simulink model "ProcessNetworkSimulation"  (R2015b)
settings: Solver=VariableStepAuto  StartTime=0.0  StopTime=1000.0  RelTol=1e-3
libraries: simulink x1, simeventslib x1
(part 18 of 21)

== system ProcessNetworkSimulation/Process_22/Process ==
  OUTQueue : FIFOQueue  Capacity=inf
  ProcessQueue : FIFOQueue  Capacity=Inf  StatAverageWait=on  StatAverageQueueLength=on
      settings: OutputPortMap=o2,o3
  ProcessServer : NServer  NumberOfServers=11  ServiceTimeFrom=Signal port t  StatNumberDeparted=on  StatUtilization=on
      settings: OutputPortMap=o0,o5
  ProcessTime : EventBasedRandomNumber  meanExp=0.05  minUnif=1  meanNorm=2  stdNorm=0.2  Seed=23578
  Routing : EventBasedRandomNumber  Distribution=Arbitrary discrete  valueVecDisc=[0,1,2,3,4,5,6,7,8,9,10,11,12,13,14,15,16,17,18,19,20,21,22,23,24,25,26,27,28,29,30,31,32,33,34,35,36,37,38,39,40,41,42,43]  probVecDisc=[0,0.0298,0.0085,0.0298,0.0383,0.0255,0.0085,0.0383,0.0383,0.0043,0.0298,0.0085,0.0085,0.0383,0.0424,0.0255,0.0085,0.0298,0.0298,0.0298,0.0128,0.0085,0.0085,0.0383,0.0383,0.0085,0.0213,0.0085,0.0298,0.0213,0.0085,0.034,0.0383,0.0383,0.0255,0.0128,0.0213,0.0298,0.0213,0.0128,0.0085,0.0383,0.0426,0]  Seed=26795
  read_ProcessTimer : ReadTimer  TimerTag=T_Process_22  StatAverageTimeElapsed=on
      settings: OutputPortMap=o3
  setRouting : SetAttribute  AttributeName=outputFlowNode  AttributeFrom=Signal port  EvaluatedAttributeValue={ []}
  start_ProcessTimer : StartTimer  TimerTag=T_Process_22  TimerStartedOption=Restart
  IN_Job : PMIOPort  Port=1  Side=Left
  OUT_Job : PMIOPort  Port=2  Side=Right
  wires:
  Routing/1 -> setRouting/1
  ProcessTime/1 -> ProcessServer/1
  connections:
  setRouting/LConn1 -- OUTQueue/RConn1
  IN_Job/RConn1 -- start_ProcessTimer/LConn1
  ProcessServer/RConn1 -- read_ProcessTimer/LConn1
  start_ProcessTimer/RConn1 -- ProcessQueue/LConn1
  ProcessQueue/RConn1 -- ProcessServer/LConn1
  read_ProcessTimer/RConn1 -- OUTQueue/LConn1
  OUT_Job/RConn1 -- setRouting/RConn1

== system ProcessNetworkSimulation/Process_23/Process ==
  OUTQueue : FIFOQueue  Capacity=inf
  ProcessQueue : FIFOQueue  Capacity=Inf  StatAverageWait=on  StatAverageQueueLength=on
      settings: OutputPortMap=o2,o3
  ProcessServer : NServer  NumberOfServers=12  ServiceTimeFrom=Signal port t  StatNumberDeparted=on  StatUtilization=on
      settings: OutputPortMap=o0,o5
  ProcessTime : EventBasedRandomNumber  meanExp=0.05  minUnif=1  meanNorm=2  stdNorm=0.2  Seed=30012
  Routing : EventBasedRandomNumber  Distribution=Arbitrary discrete  valueVecDisc=[0,1,2,3,4,5,6,7,8,9,10,11,12,13,14,15,16,17,18,19,20,21,22,23,24,25,26,27,28,29,30,31,32,33,34,35,36]  probVecDisc=[0,0.0413,0.0229,0.0275,0.0275,0.0092,0.0413,0.0458,0.0275,0.0321,0.0413,0.0413,0.0138,0.0367,0.0092,0.0092,0.0275,0.0413,0.0046,0.0413,0.0138,0.0229,0.0275,0.0092,0.0092,0.0275,0.0413,0.0275,0.0459,0.0459,0.0229,0.0413,0.0275,0.0275,0.0321,0.0321,0.0046]  Seed=33229
  read_ProcessTimer : ReadTimer  TimerTag=T_Process_23  StatAverageTimeElapsed=on
      settings: OutputPortMap=o3
  setRouting : SetAttribute  AttributeName=outputFlowNode  AttributeFrom=Signal port  EvaluatedAttributeValue={ []}
  start_ProcessTimer : StartTimer  TimerTag=T_Process_23  TimerStartedOption=Restart
  IN_Job : PMIOPort  Port=1  Side=Left
  OUT_Job : PMIOPort  Port=2  Side=Right
  wires:
  Routing/1 -> setRouting/1
  ProcessTime/1 -> ProcessServer/1
  connections:
  setRouting/LConn1 -- OUTQueue/RConn1
  IN_Job/RConn1 -- start_ProcessTimer/LConn1
  ProcessServer/RConn1 -- read_ProcessTimer/LConn1
  start_ProcessTimer/RConn1 -- ProcessQueue/LConn1
  ProcessQueue/RConn1 -- ProcessServer/LConn1
  read_ProcessTimer/RConn1 -- OUTQueue/LConn1
  OUT_Job/RConn1 -- setRouting/RConn1

== system ProcessNetworkSimulation/Process_24/Process ==
  OUTQueue : FIFOQueue  Capacity=inf
  ProcessQueue : FIFOQueue  Capacity=Inf  StatAverageWait=on  StatAverageQueueLength=on
      settings: OutputPortMap=o2,o3
  ProcessServer : NServer  NumberOfServers=12  ServiceTimeFrom=Signal port t  StatNumberDeparted=on  StatUtilization=on
      settings: OutputPortMap=o0,o5
  ProcessTime : EventBasedRandomNumber  meanExp=0.05  minUnif=1  meanNorm=2  stdNorm=0.2  Seed=36446
  Routing : EventBasedRandomNumber  Distribution=Arbitrary discrete  valueVecDisc=[0,1,2,3,4,5,6,7,8,9,10,11,12,13,14,15,16,17,18,19,20,21,22,23,24,25,26,27,28,29,30,31,32,33,34,35,36]  probVecDisc=[0,0.0051,0.0455,0.0152,0.0051,0.0253,0.0455,0.0354,0.0101,0.0152,0.0354,0.0455,0.0101,0.0354,0.0455,0.0152,0.0101,0.0303,0.0051,0.0101,0.0455,0.0455,0.0354,0.0494,0.0455,0.0455,0.0101,0.0253,0.0354,0.0303,0.0404,0.0354,0.0404,0.0303,0.0051,0.0354,0]  Seed=39663
  read_ProcessTimer : ReadTimer  TimerTag=T_Process_24  StatAverageTimeElapsed=on
      settings: OutputPortMap=o3
  setRouting : SetAttribute  AttributeName=outputFlowNode  AttributeFrom=Signal port  EvaluatedAttributeValue={ []}
  start_ProcessTimer : StartTimer  TimerTag=T_Process_24  TimerStartedOption=Restart
  IN_Job : PMIOPort  Port=1  Side=Left
  OUT_Job : PMIOPort  Port=2  Side=Right
  wires:
  Routing/1 -> setRouting/1
  ProcessTime/1 -> ProcessServer/1
  connections:
  setRouting/LConn1 -- OUTQueue/RConn1
  IN_Job/RConn1 -- start_ProcessTimer/LConn1
  ProcessServer/RConn1 -- read_ProcessTimer/LConn1
  start_ProcessTimer/RConn1 -- ProcessQueue/LConn1
  ProcessQueue/RConn1 -- ProcessServer/LConn1
  read_ProcessTimer/RConn1 -- OUTQueue/LConn1
  OUT_Job/RConn1 -- setRouting/RConn1

== system ProcessNetworkSimulation/Process_25/Process ==
  OUTQueue : FIFOQueue  Capacity=inf
  ProcessQueue : FIFOQueue  Capacity=Inf  StatAverageWait=on  StatAverageQueueLength=on
      settings: OutputPortMap=o2,o3
  ProcessServer : NServer  NumberOfServers=11  ServiceTimeFrom=Signal port t  StatNumberDeparted=on  StatUtilization=on
      settings: OutputPortMap=o0,o5
  ProcessTime : EventBasedRandomNumber  meanExp=0.05  minUnif=1  meanNorm=2  stdNorm=0.2  Seed=42880
  Routing : EventBasedRandomNumber  Distribution=Arbitrary discrete  valueVecDisc=[0,1,2,3,4,5,6,7,8,9,10,11,12,13,14,15,16,17,18,19,20,21,22,23,24,25,26,27,28,29,30,31,32,33,34,35,36,37,38,39,40,41]  probVecDisc=[0,0.0323,0.023,0.0092,0.0092,0.0415,0.023,0.0046,0.0462,0.0092,0.0461,0.0092,0.023,0.0323,0.0323,0.0323,0.0138,0.0092,0.0415,0.0138,0.0415,0.0092,0.0276,0.023,0.0323,0.023,0.0415,0.0092,0.0415,0.0046,0.0461,0.0415,0.0369,0.023,0.023,0.023,0.0046,0.0461,0.0323,0.0092,0.0092,0]  Seed=46097
  read_ProcessTimer : ReadTimer  TimerTag=T_Process_25  StatAverageTimeElapsed=on
      settings: OutputPortMap=o3
  setRouting : SetAttribute  AttributeName=outputFlowNode  AttributeFrom=Signal port  EvaluatedAttributeValue={ []}
  start_ProcessTimer : StartTimer  TimerTag=T_Process_25  TimerStartedOption=Restart
  IN_Job : PMIOPort  Port=1  Side=Left
  OUT_Job : PMIOPort  Port=2  Side=Right
  wires:
  Routing/1 -> setRouting/1
  ProcessTime/1 -> ProcessServer/1
  connections:
  setRouting/LConn1 -- OUTQueue/RConn1
  IN_Job/RConn1 -- start_ProcessTimer/LConn1
  ProcessServer/RConn1 -- read_ProcessTimer/LConn1
  start_ProcessTimer/RConn1 -- ProcessQueue/LConn1
  ProcessQueue/RConn1 -- ProcessServer/LConn1
  read_ProcessTimer/RConn1 -- OUTQueue/LConn1
  OUT_Job/RConn1 -- setRouting/RConn1

== system ProcessNetworkSimulation/Process_26/Process ==
  OUTQueue : FIFOQueue  Capacity=inf
  ProcessQueue : FIFOQueue  Capacity=Inf  StatAverageWait=on  StatAverageQueueLength=on
      settings: OutputPortMap=o2,o3
  ProcessServer : NServer  NumberOfServers=12  ServiceTimeFrom=Signal port t  StatNumberDeparted=on  StatUtilization=on
      settings: OutputPortMap=o0,o5
  ProcessTime : EventBasedRandomNumber  meanExp=0.05  minUnif=1  meanNorm=2  stdNorm=0.2  Seed=49314
  Routing : EventBasedRandomNumber  Distribution=Arbitrary discrete  valueVecDisc=[0,1,2,3,4,5,6,7,8,9,10,11,12,13,14,15,16,17,18,19,20,21,22,23,24,25,26,27,28,29,30,31,32,33,34,35,36,37,38,39,40]  probVecDisc=[0,0.0457,0.0406,0.0152,0.0102,0.0102,0.0102,0.0102,0.0254,0.0457,0.0499,0.0355,0.0102,0.0102,0.0406,0.0102,0.0355,0.0051,0.0457,0.0102,0.0152,0.0051,0.0254,0.0457,0.0102,0.0406,0.0305,0.0508,0.0457,0.0254,0.0102,0.0051,0.0355,0.0102,0.0305,0.0102,0.0102,0.0457,0.0102,0.0254,0.0457]  Seed=52531
  read_ProcessTimer : ReadTimer  TimerTag=T_Process_26  StatAverageTimeElapsed=on
      settings: OutputPortMap=o3
  setRouting : SetAttribute  AttributeName=outputFlowNode  AttributeFrom=Signal port  EvaluatedAttributeValue={ []}
  start_ProcessTimer : StartTimer  TimerTag=T_Process_26  TimerStartedOption=Restart
  IN_Job : PMIOPort  Port=1  Side=Left
  OUT_Job : PMIOPort  Port=2  Side=Right
  wires:
  Routing/1 -> setRouting/1
  ProcessTime/1 -> ProcessServer/1
  connections:
  setRouting/LConn1 -- OUTQueue/RConn1
  IN_Job/RConn1 -- start_ProcessTimer/LConn1
  ProcessServer/RConn1 -- read_ProcessTimer/LConn1
  start_ProcessTimer/RConn1 -- ProcessQueue/LConn1
  ProcessQueue/RConn1 -- ProcessServer/LConn1
  read_ProcessTimer/RConn1 -- OUTQueue/LConn1
  OUT_Job/RConn1 -- setRouting/RConn1

== system ProcessNetworkSimulation/Process_27/Process ==
  OUTQueue : FIFOQueue  Capacity=inf
  ProcessQueue : FIFOQueue  Capacity=Inf  StatAverageWait=on  StatAverageQueueLength=on
      settings: OutputPortMap=o2,o3
  ProcessServer : NServer  NumberOfServers=14  ServiceTimeFrom=Signal port t  StatNumberDeparted=on  StatUtilization=on
      settings: OutputPortMap=o0,o5
  ProcessTime : EventBasedRandomNumber  meanExp=0.05  minUnif=1  meanNorm=2  stdNorm=0.2  Seed=55748
  Routing : EventBasedRandomNumber  Distribution=Arbitrary discrete  valueVecDisc=[0,1,2,3,4,5,6,7,8,9,10,11,12,13,14,15,16,17,18,19,20,21,22,23,24,25,26,27,28,29,30,31,32,33,34,35,36,37,38,39,40,41,42,43]  probVecDisc=[0,0.0353,0.0353,0.0078,0.0078,0.0078,0.0196,0.0275,0.0078,0.0275,0.0353,0.0275,0.0353,0.0275,0.0196,0.0196,0.0235,0.0275,0.0275,0.0353,0.0275,0.0353,0.0118,0.0353,0.0078,0.0275,0.0353,0.0275,0.0078,0.039,0.0235,0.0235,0.0118,0.0275,0.0118,0.0235,0.0275,0.0196,0.0314,0.0235,0.0235,0.0353,0.0078,0]  Seed=58965
  read_ProcessTimer : ReadTimer  TimerTag=T_Process_27  StatAverageTimeElapsed=on
      settings: OutputPortMap=o3
  setRouting : SetAttribute  AttributeName=outputFlowNode  AttributeFrom=Signal port  EvaluatedAttributeValue={ []}
  start_ProcessTimer : StartTimer  TimerTag=T_Process_27  TimerStartedOption=Restart
  IN_Job : PMIOPort  Port=1  Side=Left
  OUT_Job : PMIOPort  Port=2  Side=Right
  wires:
  Routing/1 -> setRouting/1
  ProcessTime/1 -> ProcessServer/1
  connections:
  setRouting/LConn1 -- OUTQueue/RConn1
  IN_Job/RConn1 -- start_ProcessTimer/LConn1
  ProcessServer/RConn1 -- read_ProcessTimer/LConn1
  start_ProcessTimer/RConn1 -- ProcessQueue/LConn1
  ProcessQueue/RConn1 -- ProcessServer/LConn1
  read_ProcessTimer/RConn1 -- OUTQueue/LConn1
  OUT_Job/RConn1 -- setRouting/RConn1

== system ProcessNetworkSimulation/Process_28/Process ==
  OUTQueue : FIFOQueue  Capacity=inf
  ProcessQueue : FIFOQueue  Capacity=Inf  StatAverageWait=on  StatAverageQueueLength=on
      settings: OutputPortMap=o2,o3
  ProcessServer : NServer  NumberOfServers=8  ServiceTimeFrom=Signal port t  StatNumberDeparted=on  StatUtilization=on
      settings: OutputPortMap=o0,o5
  ProcessTime : EventBasedRandomNumber  meanExp=0.05  minUnif=1  meanNorm=2  stdNorm=0.2  Seed=62182
  Routing : EventBasedRandomNumber  Distribution=Arbitrary discrete  valueVecDisc=[0,1,2,3,4,5,6,7,8,9,10,11,12,13,14,15,16,17,18,19,20,21,22,23,24,25,26,27,28,29]  probVecDisc=[0,0.0643,0.0143,0.0143,0.0143,0.05,0.05,0.0571,0.0571,0.0643,0.0143,0.0715,0.0357,0.05,0.0214,0.0143,0.0357,0.0643,0.0643,0.0071,0.0429,0.0357,0.0143,0.0357,0.0214,0.05,0.0143,0.0143,0.0071,0]  Seed=65399
  read_ProcessTimer : ReadTimer  TimerTag=T_Process_28  StatAverageTimeElapsed=on
      settings: OutputPortMap=o3
  setRouting : SetAttribute  AttributeName=outputFlowNode  AttributeFrom=Signal port  EvaluatedAttributeValue={ []}
  start_ProcessTimer : StartTimer  TimerTag=T_Process_28  TimerStartedOption=Restart
  IN_Job : PMIOPort  Port=1  Side=Left
  OUT_Job : PMIOPort  Port=2  Side=Right
  wires:
  Routing/1 -> setRouting/1
  ProcessTime/1 -> ProcessServer/1
  connections:
  setRouting/LConn1 -- OUTQueue/RConn1
  IN_Job/RConn1 -- start_ProcessTimer/LConn1
  ProcessServer/RConn1 -- read_ProcessTimer/LConn1
  start_ProcessTimer/RConn1 -- ProcessQueue/LConn1
  ProcessQueue/RConn1 -- ProcessServer/LConn1
  read_ProcessTimer/RConn1 -- OUTQueue/LConn1
  OUT_Job/RConn1 -- setRouting/RConn1

== system ProcessNetworkSimulation/Process_29/Process ==
  OUTQueue : FIFOQueue  Capacity=inf
  ProcessQueue : FIFOQueue  Capacity=Inf  StatAverageWait=on  StatAverageQueueLength=on
      settings: OutputPortMap=o2,o3
  ProcessServer : NServer  NumberOfServers=12  ServiceTimeFrom=Signal port t  StatNumberDeparted=on  StatUtilization=on
      settings: OutputPortMap=o0,o5
  ProcessTime : EventBasedRandomNumber  meanExp=0.05  minUnif=1  meanNorm=2  stdNorm=0.2  Seed=3080
  Routing : EventBasedRandomNumber  Distribution=Arbitrary discrete  valueVecDisc=[0,1,2,3,4,5,6,7,8,9,10,11,12,13,14,15,16,17,18,19,20,21,22,23,24,25,26,27,28,29,30,31,32,33,34,35,36,37]  probVecDisc=[0,0.0142,0.0142,0.033,0.0283,0.0425,0.0094,0.0377,0.0471,0.033,0.0047,0.0047,0.0283,0.0283,0.0377,0.0425,0.0047,0.033,0.0094,0.0425,0.0425,0.0094,0.0472,0.0283,0.0283,0.0377,0.0283,0.033,0.0236,0.033,0.0283,0.0425,0.0425,0.0142,0.0094,0.0094,0.0472,0]  Seed=6297
  read_ProcessTimer : ReadTimer  TimerTag=T_Process_29  StatAverageTimeElapsed=on
      settings: OutputPortMap=o3
  setRouting : SetAttribute  AttributeName=outputFlowNode  AttributeFrom=Signal port  EvaluatedAttributeValue={ []}
  start_ProcessTimer : StartTimer  TimerTag=T_Process_29  TimerStartedOption=Restart
  IN_Job : PMIOPort  Port=1  Side=Left
  OUT_Job : PMIOPort  Port=2  Side=Right
  wires:
  Routing/1 -> setRouting/1
  ProcessTime/1 -> ProcessServer/1
  connections:
  setRouting/LConn1 -- OUTQueue/RConn1
  IN_Job/RConn1 -- start_ProcessTimer/LConn1
  ProcessServer/RConn1 -- read_ProcessTimer/LConn1
  start_ProcessTimer/RConn1 -- ProcessQueue/LConn1
  ProcessQueue/RConn1 -- ProcessServer/LConn1
  read_ProcessTimer/RConn1 -- OUTQueue/LConn1
  OUT_Job/RConn1 -- setRouting/RConn1

== system ProcessNetworkSimulation/Process_3/Process ==
  OUTQueue : FIFOQueue  Capacity=inf
  ProcessQueue : FIFOQueue  Capacity=Inf  StatAverageWait=on  StatAverageQueueLength=on
      settings: OutputPortMap=o2,o3
  ProcessServer : NServer  NumberOfServers=10  ServiceTimeFrom=Signal port t  StatNumberDeparted=on  StatUtilization=on
      settings: OutputPortMap=o0,o5
  ProcessTime : EventBasedRandomNumber  meanExp=0.05  minUnif=1  meanNorm=2  stdNorm=0.2  Seed=9514
  Routing : EventBasedRandomNumber  Distribution=Arbitrary discrete  valueVecDisc=[0,1,2,3,4,5,6,7,8,9,10,11,12,13,14,15,16,17,18,19,20,21,22,23,24,25,26,27,28,29,30,31]  probVecDisc=[0,0.0335,0.0503,0.0503,0.0112,0.0279,0.0279,0.0503,0.0503,0.0112,0.0391,0.0557,0.0391,0.0112,0.0168,0.0503,0.0335,0.0391,0.0112,0.0335,0.0112,0.0391,0.0056,0.0279,0.0112,0.0279,0.0503,0.0503,0.0391,0.0559,0.0112,0.0279]  Seed=12731
  read_ProcessTimer : ReadTimer  TimerTag=T_Process_3  StatAverageTimeElapsed=on
      settings: OutputPortMap=o3
  setRouting : SetAttribute  AttributeName=outputFlowNode  AttributeFrom=Signal port  EvaluatedAttributeValue={ []}
  start_ProcessTimer : StartTimer  TimerTag=T_Process_3  TimerStartedOption=Restart
  IN_Job : PMIOPort  Port=1  Side=Left
  OUT_Job : PMIOPort  Port=2  Side=Right
  wires:
  Routing/1 -> setRouting/1
  ProcessTime/1 -> ProcessServer/1
  connections:
  setRouting/LConn1 -- OUTQueue/RConn1
  IN_Job/RConn1 -- start_ProcessTimer/LConn1
  ProcessServer/RConn1 -- read_ProcessTimer/LConn1
  start_ProcessTimer/RConn1 -- ProcessQueue/LConn1
  ProcessQueue/RConn1 -- ProcessServer/LConn1
  read_ProcessTimer/RConn1 -- OUTQueue/LConn1
  OUT_Job/RConn1 -- setRouting/RConn1

== system ProcessNetworkSimulation/Process_30/Process ==
  OUTQueue : FIFOQueue  Capacity=inf
  ProcessQueue : FIFOQueue  Capacity=Inf  StatAverageWait=on  StatAverageQueueLength=on
      settings: OutputPortMap=o2,o3
  ProcessServer : NServer  NumberOfServers=12  ServiceTimeFrom=Signal port t  StatNumberDeparted=on  StatUtilization=on
      settings: OutputPortMap=o0,o5
  ProcessTime : EventBasedRandomNumber  meanExp=0.05  minUnif=1  meanNorm=2  stdNorm=0.2  Seed=15948
  Routing : EventBasedRandomNumber  Distribution=Arbitrary discrete  valueVecDisc=[0,1,2,3,4,5,6,7,8,9,10,11,12,13,14,15,16,17,18,19,20,21,22,23,24,25,26,27,28,29,30,31,32,33,34,35,36,37,38]  probVecDisc=[0,0.0474,0.0316,0.0316,0.0316,0.0158,0.0527,0.0421,0.0368,0.0105,0.0316,0.0105,0.0474,0.0263,0.0316,0.0105,0.0368,0.0053,0.0158,0.0053,0.0474,0.0368,0.0105,0.0474,0.0053,0.0316,0.0105,0.0053,0.0105,0.0158,0.0526,0.0105,0.0368,0.0105,0.0263,0.0368,0.0474,0.0368,0]  Seed=19165
  read_ProcessTimer : ReadTimer  TimerTag=T_Process_30  StatAverageTimeElapsed=on
      settings: OutputPortMap=o3
  setRouting : SetAttribute  AttributeName=outputFlowNode  AttributeFrom=Signal port  EvaluatedAttributeValue={ []}
  start_ProcessTimer : StartTimer  TimerTag=T_Process_30  TimerStartedOption=Restart
  IN_Job : PMIOPort  Port=1  Side=Left
  OUT_Job : PMIOPort  Port=2  Side=Right
  wires:
  Routing/1 -> setRouting/1
  ProcessTime/1 -> ProcessServer/1
  connections:
  setRouting/LConn1 -- OUTQueue/RConn1
  IN_Job/RConn1 -- start_ProcessTimer/LConn1
  ProcessServer/RConn1 -- read_ProcessTimer/LConn1
  start_ProcessTimer/RConn1 -- ProcessQueue/LConn1
  ProcessQueue/RConn1 -- ProcessServer/LConn1
  read_ProcessTimer/RConn1 -- OUTQueue/LConn1
  OUT_Job/RConn1 -- setRouting/RConn1

== system ProcessNetworkSimulation/Process_31/Process ==
  OUTQueue : FIFOQueue  Capacity=inf
  ProcessQueue : FIFOQueue  Capacity=Inf  StatAverageWait=on  StatAverageQueueLength=on
      settings: OutputPortMap=o2,o3
  ProcessServer : NServer  NumberOfServers=9  ServiceTimeFrom=Signal port t  StatNumberDeparted=on  StatUtilization=on
      settings: OutputPortMap=o0,o5
  ProcessTime : EventBasedRandomNumber  meanExp=0.05  minUnif=1  meanNorm=2  stdNorm=0.2  Seed=22382
  Routing : EventBasedRandomNumber  Distribution=Arbitrary discrete  valueVecDisc=[0,1,2,3,4,5,6,7,8,9,10,11,12,13,14,15,16,17,18,19,20,21,22,23,24,25,26,27,28]  probVecDisc=[0,0.0071,0.0142,0.0496,0.0638,0.0638,0.0355,0.0142,0.0496,0.0426,0.0071,0.0355,0.0638,0.0426,0.0426,0.0707,0.0638,0.0213,0.0142,0.0213,0.0213,0.0071,0.0142,0.0071,0.0426,0.0426,0.0638,0.0142,0.0638]  Seed=25599
  read_ProcessTimer : ReadTimer  TimerTag=T_Process_31  StatAverageTimeElapsed=on
      settings: OutputPortMap=o3
  setRouting : SetAttribute  AttributeName=outputFlowNode  AttributeFrom=Signal port  EvaluatedAttributeValue={ []}
  start_ProcessTimer : StartTimer  TimerTag=T_Process_31  TimerStartedOption=Restart
  IN_Job : PMIOPort  Port=1  Side=Left
  OUT_Job : PMIOPort  Port=2  Side=Right
  wires:
  Routing/1 -> setRouting/1
  ProcessTime/1 -> ProcessServer/1
  connections:
  setRouting/LConn1 -- OUTQueue/RConn1
  IN_Job/RConn1 -- start_ProcessTimer/LConn1
  ProcessServer/RConn1 -- read_ProcessTimer/LConn1
  start_ProcessTimer/RConn1 -- ProcessQueue/LConn1
  ProcessQueue/RConn1 -- ProcessServer/LConn1
  read_ProcessTimer/RConn1 -- OUTQueue/LConn1
  OUT_Job/RConn1 -- setRouting/RConn1

== system ProcessNetworkSimulation/Process_32/Process ==
  OUTQueue : FIFOQueue  Capacity=inf
  ProcessQueue : FIFOQueue  Capacity=Inf  StatAverageWait=on  StatAverageQueueLength=on
      settings: OutputPortMap=o2,o3
  ProcessServer : NServer  NumberOfServers=10  ServiceTimeFrom=Signal port t  StatNumberDeparted=on  StatUtilization=on
      settings: OutputPortMap=o0,o5
  ProcessTime : EventBasedRandomNumber  meanExp=0.05  minUnif=1  meanNorm=2  stdNorm=0.2  Seed=28816
  Routing : EventBasedRandomNumber  Distribution=Arbitrary discrete  valueVecDisc=[0,1,2,3,4,5,6,7,8,9,10,11,12,13,14,15,16,17,18,19,20,21,22,23,24,25,26,27,28,29,30,31,32,33,34,35,36,37,38]  probVecDisc=[0,0.0114,0.0284,0.0564,0.0114,0.0398,0.0284,0.0284,0.0114,0.0114,0.0114,0.017,0.0284,0.0398,0.0114,0.0455,0.0511,0.0284,0.0398,0.0398,0.0114,0.0398,0.0511,0.0114,0.0114,0.0284,0.0114,0.0284,0.017,0.0398,0.0284,0.0114,0.0398,0.0341,0.0284,0.0114,0.0398,0.017,0]  Seed=32033
  read_ProcessTimer : ReadTimer  TimerTag=T_Process_32  StatAverageTimeElapsed=on
      settings: OutputPortMap=o3
  setRouting : SetAttribute  AttributeName=outputFlowNode  AttributeFrom=Signal port  EvaluatedAttributeValue={ []}
  start_ProcessTimer : StartTimer  TimerTag=T_Process_32  TimerStartedOption=Restart
  IN_Job : PMIOPort  Port=1  Side=Left
  OUT_Job : PMIOPort  Port=2  Side=Right
  wires:
  Routing/1 -> setRouting/1
  ProcessTime/1 -> ProcessServer/1
  connections:
  setRouting/LConn1 -- OUTQueue/RConn1
  IN_Job/RConn1 -- start_ProcessTimer/LConn1
  ProcessServer/RConn1 -- read_ProcessTimer/LConn1
  start_ProcessTimer/RConn1 -- ProcessQueue/LConn1
  ProcessQueue/RConn1 -- ProcessServer/LConn1
  read_ProcessTimer/RConn1 -- OUTQueue/LConn1
  OUT_Job/RConn1 -- setRouting/RConn1

== system ProcessNetworkSimulation/Process_33/Process ==
  OUTQueue : FIFOQueue  Capacity=inf
  ProcessQueue : FIFOQueue  Capacity=Inf  StatAverageWait=on  StatAverageQueueLength=on
      settings: OutputPortMap=o2,o3
  ProcessServer : NServer  NumberOfServers=11  ServiceTimeFrom=Signal port t  StatNumberDeparted=on  StatUtilization=on
      settings: OutputPortMap=o0,o5
  ProcessTime : EventBasedRandomNumber  meanExp=0.05  minUnif=1  meanNorm=2  stdNorm=0.2  Seed=35250
  Routing : EventBasedRandomNumber  Distribution=Arbitrary discrete  valueVecDisc=[0,1,2,3,4,5,6,7,8,9,10,11,12,13,14,15,16,17,18,19,20,21,22,23,24,25,26,27,28,29,30,31,32,33,34,35,36,37,38,39,40,41,42]  probVecDisc=[0,0.0101,0.0446,0.0151,0.0452,0.0452,0.0101,0.0452,0.0101,0.0151,0.0452,0.0452,0.0251,0.0352,0.0101,0.0151,0.0352,0.0151,0.0352,0.0302,0.0352,0.0101,0.005,0.0101,0.0452,0.0101,0.0251,0.0101,0.0101,0.0302,0.0251,0.0251,0.0452,0.0101,0.005,0.0101,0.0101,0.0101,0.0251,0.0302,0.0452,0.0352,0]  Seed=38467
  read_ProcessTimer : ReadTimer  TimerTag=T_Process_33  StatAverageTimeElapsed=on
      settings: OutputPortMap=o3
  setRouting : SetAttribute  AttributeName=outputFlowNode  AttributeFrom=Signal port  EvaluatedAttributeValue={ []}
  start_ProcessTimer : StartTimer  TimerTag=T_Process_33  TimerStartedOption=Restart
  IN_Job : PMIOPort  Port=1  Side=Left
  OUT_Job : PMIOPort  Port=2  Side=Right
  wires:
  Routing/1 -> setRouting/1
  ProcessTime/1 -> ProcessServer/1
  connections:
  setRouting/LConn1 -- OUTQueue/RConn1
  IN_Job/RConn1 -- start_ProcessTimer/LConn1
  ProcessServer/RConn1 -- read_ProcessTimer/LConn1
  start_ProcessTimer/RConn1 -- ProcessQueue/LConn1
  ProcessQueue/RConn1 -- ProcessServer/LConn1
  read_ProcessTimer/RConn1 -- OUTQueue/LConn1
  OUT_Job/RConn1 -- setRouting/RConn1

== system ProcessNetworkSimulation/Process_34/Process ==
  OUTQueue : FIFOQueue  Capacity=inf
  ProcessQueue : FIFOQueue  Capacity=Inf  StatAverageWait=on  StatAverageQueueLength=on
      settings: OutputPortMap=o2,o3
  ProcessServer : NServer  NumberOfServers=11  ServiceTimeFrom=Signal port t  StatNumberDeparted=on  StatUtilization=on
      settings: OutputPortMap=o0,o5
  ProcessTime : EventBasedRandomNumber  meanExp=0.05  minUnif=1  meanNorm=2  stdNorm=0.2  Seed=41684
  Routing : EventBasedRandomNumber  Distribution=Arbitrary discrete  valueVecDisc=[0,1,2,3,4,5,6,7,8,9,10,11,12,13,14,15,16,17,18,19,20,21,22,23,24,25,26,27,28,29,30,31,32,33,34,35,36,37,38,39,40]  probVecDisc=[0,0.0259,0.0129,0.0302,0.0086,0.0216,0.0129,0.0302,0.0129,0.0345,0.0345,0.0388,0.0259,0.0216,0.0302,0.0086,0.0216,0.0086,0.0086,0.0302,0.0424,0.0259,0.0388,0.0259,0.0302,0.0302,0.0086,0.0259,0.0388,0.0302,0.0216,0.0129,0.0216,0.0302,0.0216,0.0259,0.0302,0.0431,0.0216,0.0259,0.0302]  Seed=44901
  read_ProcessTimer : ReadTimer  TimerTag=T_Process_34  StatAverageTimeElapsed=on
      settings: OutputPortMap=o3
  setRouting : SetAttribute  AttributeName=outputFlowNode  AttributeFrom=Signal port  EvaluatedAttributeValue={ []}
  start_ProcessTimer : StartTimer  TimerTag=T_Process_34  TimerStartedOption=Restart
  IN_Job : PMIOPort  Port=1  Side=Left
  OUT_Job : PMIOPort  Port=2  Side=Right
  wires:
  Routing/1 -> setRouting/1
  ProcessTime/1 -> ProcessServer/1
  connections:
  setRouting/LConn1 -- OUTQueue/RConn1
  IN_Job/RConn1 -- start_ProcessTimer/LConn1
  ProcessServer/RConn1 -- read_ProcessTimer/LConn1
  start_ProcessTimer/RConn1 -- ProcessQueue/LConn1
  ProcessQueue/RConn1 -- ProcessServer/LConn1
  read_ProcessTimer/RConn1 -- OUTQueue/LConn1
  OUT_Job/RConn1 -- setRouting/RConn1

== system ProcessNetworkSimulation/Process_35/Process ==
  OUTQueue : FIFOQueue  Capacity=inf
  ProcessQueue : FIFOQueue  Capacity=Inf  StatAverageWait=on  StatAverageQueueLength=on
      settings: OutputPortMap=o2,o3
  ProcessServer : NServer  NumberOfServers=12  ServiceTimeFrom=Signal port t  StatNumberDeparted=on  StatUtilization=on
      settings: OutputPortMap=o0,o5
  ProcessTime : EventBasedRandomNumber  meanExp=0.05  minUnif=1  meanNorm=2  stdNorm=0.2  Seed=48118
  Routing : EventBasedRandomNumber  Distribution=Arbitrary discrete  valueVecDisc=[0,1,2,3,4,5,6,7,8,9,10,11,12,13,14,15,16,17,18,19,20,21,22,23,24,25,26,27,28,29,30,31,32,33,34,35,36,37,38]  probVecDisc=[0,0.0133,0.04,0.0311,0.0222,0.04,0.0089,0.04,0.0445,0.0089,0.0267,0.0267,0.0222,0.0222,0.0089,0.0267,0.0089,0.04,0.0133,0.04,0.0222,0.0089,0.0267,0.0089,0.0089,0.0267,0.0133,0.0222,0.0444,0.0444,0.04,0.0222,0.0222,0.0267,0.0356,0.0311,0.0311,0.04,0.04]  Seed=51335
  read_ProcessTimer : ReadTimer  TimerTag=T_Process_35  StatAverageTimeElapsed=on
      settings: OutputPortMap=o3
  setRouting : SetAttribute  AttributeName=outputFlowNode  AttributeFrom=Signal port  EvaluatedAttributeValue={ []}
  start_ProcessTimer : StartTimer  TimerTag=T_Process_35  TimerStartedOption=Restart
  IN_Job : PMIOPort  Port=1  Side=Left
  OUT_Job : PMIOPort  Port=2  Side=Right
  wires:
  Routing/1 -> setRouting/1
  ProcessTime/1 -> ProcessServer/1
  connections:
  setRouting/LConn1 -- OUTQueue/RConn1
  IN_Job/RConn1 -- start_ProcessTimer/LConn1
  ProcessServer/RConn1 -- read_ProcessTimer/LConn1
  start_ProcessTimer/RConn1 -- ProcessQueue/LConn1
  ProcessQueue/RConn1 -- ProcessServer/LConn1
  read_ProcessTimer/RConn1 -- OUTQueue/LConn1
  OUT_Job/RConn1 -- setRouting/RConn1

== system ProcessNetworkSimulation/Process_36/Process ==
  OUTQueue : FIFOQueue  Capacity=inf
  ProcessQueue : FIFOQueue  Capacity=Inf  StatAverageWait=on  StatAverageQueueLength=on
      settings: OutputPortMap=o2,o3
  ProcessServer : NServer  NumberOfServers=11  ServiceTimeFrom=Signal port t  StatNumberDeparted=on  StatUtilization=on
      settings: OutputPortMap=o0,o5
  ProcessTime : EventBasedRandomNumber  meanExp=0.05  minUnif=1  meanNorm=2  stdNorm=0.2  Seed=54552
  Routing : EventBasedRandomNumber  Distribution=Arbitrary discrete  valueVecDisc=[0,1,2,3,4,5,6,7,8,9,10,11,12,13,14,15,16,17,18,19,20,21,22,23,24,25,26,27,28,29,30,31,32,33,34,35,36]  probVecDisc=[0,0.0374,0.0107,0.0321,0.0267,0.0374,0.0428,0.0267,0.0107,0.0374,0.0321,0.0374,0.0539,0.0321,0.016,0.0107,0.0428,0.0481,0.0374,0.0107,0.0107,0.0374,0.0481,0.0374,0.0107,0.0107,0.0374,0.0374,0.0321,0.0107,0.0107,0.0481,0.0107,0.0107,0.0481,0.016,0]  Seed=57769
  read_ProcessTimer : ReadTimer  TimerTag=T_Process_36  StatAverageTimeElapsed=on
      settings: OutputPortMap=o3
  setRouting : SetAttribute  AttributeName=outputFlowNode  AttributeFrom=Signal port  EvaluatedAttributeValue={ []}
  start_ProcessTimer : StartTimer  TimerTag=T_Process_36  TimerStartedOption=Restart
  IN_Job : PMIOPort  Port=1  Side=Left
  OUT_Job : PMIOPort  Port=2  Side=Right
  wires:
  Routing/1 -> setRouting/1
  ProcessTime/1 -> ProcessServer/1
  connections:
  setRouting/LConn1 -- OUTQueue/RConn1
  IN_Job/RConn1 -- start_ProcessTimer/LConn1
  ProcessServer/RConn1 -- read_ProcessTimer/LConn1
  start_ProcessTimer/RConn1 -- ProcessQueue/LConn1
  ProcessQueue/RConn1 -- ProcessServer/LConn1
  read_ProcessTimer/RConn1 -- OUTQueue/LConn1
  OUT_Job/RConn1 -- setRouting/RConn1

== system ProcessNetworkSimulation/Process_37/Process ==
  OUTQueue : FIFOQueue  Capacity=inf
  ProcessQueue : FIFOQueue  Capacity=Inf  StatAverageWait=on  StatAverageQueueLength=on
      settings: OutputPortMap=o2,o3
  ProcessServer : NServer  NumberOfServers=10  ServiceTimeFrom=Signal port t  StatNumberDeparted=on  StatUtilization=on
      settings: OutputPortMap=o0,o5
  ProcessTime : EventBasedRandomNumber  meanExp=0.05  minUnif=1  meanNorm=2  stdNorm=0.2  Seed=60986
  Routing : EventBasedRandomNumber  Distribution=Arbitrary discrete  valueVecDisc=[0,1,2,3,4,5,6,7,8,9,10,11,12,13,14,15,16,17,18,19,20,21,22,23,24,25,26,27,28,29,30,31,32,33,34,35]  probVecDisc=[0,0.0393,0.0281,0.0112,0.0281,0.0506,0.0506,0.0112,0.0393,0.0449,0.0112,0.0506,0.0112,0.0337,0.0281,0.0506,0.0056,0.0449,0.0169,0.0112,0.0281,0.0112,0.0112,0.0393,0.0056,0.0169,0.0112,0.0112,0.0564,0.0337,0.0337,0.0506,0.0337,0.0393,0.0506,0]  Seed=64203
  read_ProcessTimer : ReadTimer  TimerTag=T_Process_37  StatAverageTimeElapsed=on
      settings: OutputPortMap=o3
  setRouting : SetAttribute  AttributeName=outputFlowNode  AttributeFrom=Signal port  EvaluatedAttributeValue={ []}
  start_ProcessTimer : StartTimer  TimerTag=T_Process_37  TimerStartedOption=Restart
  IN_Job : PMIOPort  Port=1  Side=Left
  OUT_Job : PMIOPort  Port=2  Side=Right
  wires:
  Routing/1 -> setRouting/1
  ProcessTime/1 -> ProcessServer/1
  connections:
  setRouting/LConn1 -- OUTQueue/RConn1
  IN_Job/RConn1 -- start_ProcessTimer/LConn1
  ProcessServer/RConn1 -- read_ProcessTimer/LConn1
  start_ProcessTimer/RConn1 -- ProcessQueue/LConn1
  ProcessQueue/RConn1 -- ProcessServer/LConn1
  read_ProcessTimer/RConn1 -- OUTQueue/LConn1
  OUT_Job/RConn1 -- setRouting/RConn1

== system ProcessNetworkSimulation/Process_38/Process ==
  OUTQueue : FIFOQueue  Capacity=inf
  ProcessQueue : FIFOQueue  Capacity=Inf  StatAverageWait=on  StatAverageQueueLength=on
      settings: OutputPortMap=o2,o3
  ProcessServer : NServer  NumberOfServers=13  ServiceTimeFrom=Signal port t  StatNumberDeparted=on  StatUtilization=on
      settings: OutputPortMap=o0,o5
  ProcessTime : EventBasedRandomNumber  meanExp=0.05  minUnif=1  meanNorm=2  stdNorm=0.2  Seed=1884
  Routing : EventBasedRandomNumber  Distribution=Arbitrary discrete  valueVecDisc=[0,1,2,3,4,5,6,7,8,9,10,11,12,13,14,15,16,17,18,19,20,21,22,23,24,25,26,27,28,29,30,31,32,33,34,35,36,37,38]  probVecDisc=[0,0.0136,0.0271,0.0226,0.009,0.0136,0.0413,0.0407,0.0407,0.0271,0.0317,0.0407,0.0407,0.0317,0.0407,0.0317,0.0226,0.0407,0.0271,0.0226,0.0226,0.0317,0.0407,0.0407,0.0136,0.0317,0.0271,0.0045,0.0317,0.0407,0.009,0.0226,0.0226,0.009,0.009,0.0226,0.0226,0.0317,0]  Seed=5101
  read_ProcessTimer : ReadTimer  TimerTag=T_Process_38  StatAverageTimeElapsed=on
      settings: OutputPortMap=o3
  setRouting : SetAttribute  AttributeName=outputFlowNode  AttributeFrom=Signal port  EvaluatedAttributeValue={ []}
  start_ProcessTimer : StartTimer  TimerTag=T_Process_38  TimerStartedOption=Restart
  IN_Job : PMIOPort  Port=1  Side=Left
  OUT_Job : PMIOPort  Port=2  Side=Right
  wires:
  Routing/1 -> setRouting/1
  ProcessTime/1 -> ProcessServer/1
  connections:
  setRouting/LConn1 -- OUTQueue/RConn1
  IN_Job/RConn1 -- start_ProcessTimer/LConn1
  ProcessServer/RConn1 -- read_ProcessTimer/LConn1
  start_ProcessTimer/RConn1 -- ProcessQueue/LConn1
  ProcessQueue/RConn1 -- ProcessServer/LConn1
  read_ProcessTimer/RConn1 -- OUTQueue/LConn1
  OUT_Job/RConn1 -- setRouting/RConn1

== system ProcessNetworkSimulation/Process_39/Process ==
  OUTQueue : FIFOQueue  Capacity=inf
  ProcessQueue : FIFOQueue  Capacity=Inf  StatAverageWait=on  StatAverageQueueLength=on
      settings: OutputPortMap=o2,o3
  ProcessServer : NServer  NumberOfServers=11  ServiceTimeFrom=Signal port t  StatNumberDeparted=on  StatUtilization=on
      settings: OutputPortMap=o0,o5
  ProcessTime : EventBasedRandomNumber  meanExp=0.05  minUnif=1  meanNorm=2  stdNorm=0.2  Seed=8318
  Routing : EventBasedRandomNumber  Distribution=Arbitrary discrete  valueVecDisc=[0,1,2,3,4,5,6,7,8,9,10,11,12,13,14,15,16,17,18,19,20,21,22,23,24,25,26,27,28,29,30,31,32,33,34,35,36,37,38]  probVecDisc=[0,0.0088,0.0395,0.0307,0.0219,0.0307,0.0132,0.0307,0.0307,0.0088,0.0263,0.0395,0.0307,0.0088,0.0219,0.0263,0.0219,0.0351,0.0395,0.0435,0.0307,0.0439,0.0088,0.0395,0.0395,0.0307,0.0307,0.0395,0.0088,0.0219,0.0351,0.0088,0.0351,0.0263,0.0395,0.0132,0.0088,0.0307,0]  Seed=11535
  read_ProcessTimer : ReadTimer  TimerTag=T_Process_39  StatAverageTimeElapsed=on
      settings: OutputPortMap=o3
  setRouting : SetAttribute  AttributeName=outputFlowNode  AttributeFrom=Signal port  EvaluatedAttributeValue={ []}
  start_ProcessTimer : StartTimer  TimerTag=T_Process_39  TimerStartedOption=Restart
  IN_Job : PMIOPort  Port=1  Side=Left
  OUT_Job : PMIOPort  Port=2  Side=Right
  wires:
  Routing/1 -> setRouting/1
  ProcessTime/1 -> ProcessServer/1
  connections:
  setRouting/LConn1 -- OUTQueue/RConn1
  IN_Job/RConn1 -- start_ProcessTimer/LConn1
  ProcessServer/RConn1 -- read_ProcessTimer/LConn1
  start_ProcessTimer/RConn1 -- ProcessQueue/LConn1
  ProcessQueue/RConn1 -- ProcessServer/LConn1
  read_ProcessTimer/RConn1 -- OUTQueue/LConn1
  OUT_Job/RConn1 -- setRouting/RConn1

== system ProcessNetworkSimulation/Process_4/Process ==
  OUTQueue : FIFOQueue  Capacity=inf
  ProcessQueue : FIFOQueue  Capacity=Inf  StatAverageWait=on  StatAverageQueueLength=on
      settings: OutputPortMap=o2,o3
  ProcessServer : NServer  NumberOfServers=13  ServiceTimeFrom=Signal port t  StatNumberDeparted=on  StatUtilization=on
      settings: OutputPortMap=o0,o5
  ProcessTime : EventBasedRandomNumber  meanExp=0.05  minUnif=1  meanNorm=2  stdNorm=0.2  Seed=14752
  Routing : EventBasedRandomNumber  Distribution=Arbitrary discrete  valueVecDisc=[0,1,2,3,4,5,6,7,8,9,10,11,12,13,14,15,16,17,18,19,20,21,22,23,24,25,26,27,28,29,30,31,32,33,34,35,36,37]  probVecDisc=[0,0.0108,0.0269,0.0376,0.0532,0.0484,0.043,0.0054,0.0376,0.0108,0.0161,0.0108,0.0484,0.0269,0.0484,0.0108,0.0161,0.0538,0.0108,0.0484,0.0484,0.043,0.0269,0.0108,0.0269,0.0161,0.0108,0.0484,0.0108,0.0108,0.0054,0.0376,0.0376,0.0484,0.0108,0.0108,0.0323,0]  Seed=17969
  read_ProcessTimer : ReadTimer  TimerTag=T_Process_4  StatAverageTimeElapsed=on
      settings: OutputPortMap=o3
  setRouting : SetAttribute  AttributeName=outputFlowNode  AttributeFrom=Signal port  EvaluatedAttributeValue={ []}
  start_ProcessTimer : StartTimer  TimerTag=T_Process_4  TimerStartedOption=Restart
  IN_Job : PMIOPort  Port=1  Side=Left
  OUT_Job : PMIOPort  Port=2  Side=Right
  wires:
  Routing/1 -> setRouting/1
  ProcessTime/1 -> ProcessServer/1
  connections:
  setRouting/LConn1 -- OUTQueue/RConn1
  IN_Job/RConn1 -- start_ProcessTimer/LConn1
  ProcessServer/RConn1 -- read_ProcessTimer/LConn1
  start_ProcessTimer/RConn1 -- ProcessQueue/LConn1
  ProcessQueue/RConn1 -- ProcessServer/LConn1
  read_ProcessTimer/RConn1 -- OUTQueue/LConn1
  OUT_Job/RConn1 -- setRouting/RConn1

== system ProcessNetworkSimulation/Process_40/Process ==
  OUTQueue : FIFOQueue  Capacity=inf
  ProcessQueue : FIFOQueue  Capacity=Inf  StatAverageWait=on  StatAverageQueueLength=on
      settings: OutputPortMap=o2,o3
  ProcessServer : NServer  NumberOfServers=14  ServiceTimeFrom=Signal port t  StatNumberDeparted=on  StatUtilization=on
      settings: OutputPortMap=o0,o5
  ProcessTime : EventBasedRandomNumber  meanExp=0.05  minUnif=1  meanNorm=2  stdNorm=0.2  Seed=21186
  Routing : EventBasedRandomNumber  Distribution=Arbitrary discrete  valueVecDisc=[0,1,2,3,4,5,6,7,8,9,10,11,12,13,14,15,16,17,18,19,20,21,22,23,24,25,26,27,28,29,30,31,32,33,34,35,36,37,38,39,40,41,42,43,44,45]  probVecDisc=[0,0.0236,0.0353,0.0354,0.0236,0.0276,0.0079,0.0236,0.0236,0.0079,0.0236,0.0354,0.0276,0.0276,0.0118,0.0236,0.0276,0.0276,0.0276,0.0236,0.0276,0.0197,0.0197,0.0354,0.0315,0.0118,0.0276,0.0079,0.0276,0.0276,0.0236,0.0039,0.0079,0.0236,0.0354,0.0354,0.0236,0.0276,0.0118,0.0079,0.0079,0.0354,0.0039,0.0276,0.0236,0]  Seed=24403
  read_ProcessTimer : ReadTimer  TimerTag=T_Process_40  StatAverageTimeElapsed=on
      settings: OutputPortMap=o3
  setRouting : SetAttribute  AttributeName=outputFlowNode  AttributeFrom=Signal port  EvaluatedAttributeValue={ []}
  start_ProcessTimer : StartTimer  TimerTag=T_Process_40  TimerStartedOption=Restart
  IN_Job : PMIOPort  Port=1  Side=Left
  OUT_Job : PMIOPort  Port=2  Side=Right
  wires:
  Routing/1 -> setRouting/1
  ProcessTime/1 -> ProcessServer/1
  connections:
  setRouting/LConn1 -- OUTQueue/RConn1
  IN_Job/RConn1 -- start_ProcessTimer/LConn1
  ProcessServer/RConn1 -- read_ProcessTimer/LConn1
  start_ProcessTimer/RConn1 -- ProcessQueue/LConn1
  ProcessQueue/RConn1 -- ProcessServer/LConn1
  read_ProcessTimer/RConn1 -- OUTQueue/LConn1
  OUT_Job/RConn1 -- setRouting/RConn1

== system ProcessNetworkSimulation/Process_41/Process ==
  OUTQueue : FIFOQueue  Capacity=inf
  ProcessQueue : FIFOQueue  Capacity=Inf  StatAverageWait=on  StatAverageQueueLength=on
      settings: OutputPortMap=o2,o3
  ProcessServer : NServer  NumberOfServers=16  ServiceTimeFrom=Signal port t  StatNumberDeparted=on  StatUtilization=on
      settings: OutputPortMap=o0,o5
  ProcessTime : EventBasedRandomNumber  meanExp=0.05  minUnif=1  meanNorm=2  stdNorm=0.2  Seed=27620
  Routing : EventBasedRandomNumber  Distribution=Arbitrary discrete  valueVecDisc=[0,1,2,3,4,5,6,7,8,9,10,11,12,13,14,15,16,17,18,19,20,21,22,23,24,25,26,27,28,29,30,31,32,33,34,35,36,37,38,39,40,41,42,43,44,45,46,47]  probVecDisc=[0,0.0068,0.0068,0.0307,0.0307,0.0273,0.0102,0.0273,0.0171,0.0205,0.0239,0.0342,0.0034,0.0205,0.0239,0.0239,0.0307,0.0307,0.0307,0.0307,0.0068,0.0171,0.0273,0.0205,0.0341,0.0239,0.0068,0.0239,0.0102,0.0171,0.0239,0.0239,0.0239,0.0341,0.0205,0.0307,0.0239,0.0341,0.0068,0.0171,0.0307,0.0171,0.0171,0.0068,0.0171,0.0239,0.0307,0]  Seed=30837
  read_ProcessTimer : ReadTimer  TimerTag=T_Process_41  StatAverageTimeElapsed=on
      settings: OutputPortMap=o3
  setRouting : SetAttribute  AttributeName=outputFlowNode  AttributeFrom=Signal port  EvaluatedAttributeValue={ []}
  start_ProcessTimer : StartTimer  TimerTag=T_Process_41  TimerStartedOption=Restart
  IN_Job : PMIOPort  Port=1  Side=Left
  OUT_Job : PMIOPort  Port=2  Side=Right
  wires:
  Routing/1 -> setRouting/1
  ProcessTime/1 -> ProcessServer/1
  connections:
  setRouting/LConn1 -- OUTQueue/RConn1
  IN_Job/RConn1 -- start_ProcessTimer/LConn1
  ProcessServer/RConn1 -- read_ProcessTimer/LConn1
  start_ProcessTimer/RConn1 -- ProcessQueue/LConn1
  ProcessQueue/RConn1 -- ProcessServer/LConn1
  read_ProcessTimer/RConn1 -- OUTQueue/LConn1
  OUT_Job/RConn1 -- setRouting/RConn1

== system ProcessNetworkSimulation/Process_42/Process ==
  OUTQueue : FIFOQueue  Capacity=inf
  ProcessQueue : FIFOQueue  Capacity=Inf  StatAverageWait=on  StatAverageQueueLength=on
      settings: OutputPortMap=o2,o3
  ProcessServer : NServer  NumberOfServers=12  ServiceTimeFrom=Signal port t  StatNumberDeparted=on  StatUtilization=on
      settings: OutputPortMap=o0,o5
  ProcessTime : EventBasedRandomNumber  meanExp=0.05  minUnif=1  meanNorm=2  stdNorm=0.2  Seed=34054
  Routing : EventBasedRandomNumber  Distribution=Arbitrary discrete  valueVecDisc=[0,1,2,3,4,5,6,7,8,9,10,11,12,13,14,15,16,17,18,19,20,21,22,23,24,25,26,27,28,29,30,31,32,33,34,35]  probVecDisc=[0,0.0415,0.0415,0.023,0.0276,0.0415,0.0092,0.0464,0.0415,0.0323,0.0092,0.023,0.0323,0.0276,0.0461,0.0138,0.0138,0.0138,0.0415,0.0138,0.023,0.0323,0.0276,0.0415,0.0276,0.0276,0.0276,0.0276,0.0415,0.0369,0.0276,0.023,0.023,0.0415,0.0323,0]  Seed=37271
  read_ProcessTimer : ReadTimer  TimerTag=T_Process_42  StatAverageTimeElapsed=on
      settings: OutputPortMap=o3
  setRouting : SetAttribute  AttributeName=outputFlowNode  AttributeFrom=Signal port  EvaluatedAttributeValue={ []}
  start_ProcessTimer : StartTimer  TimerTag=T_Process_42  TimerStartedOption=Restart
  IN_Job : PMIOPort  Port=1  Side=Left
  OUT_Job : PMIOPort  Port=2  Side=Right
  wires:
  Routing/1 -> setRouting/1
  ProcessTime/1 -> ProcessServer/1
  connections:
  setRouting/LConn1 -- OUTQueue/RConn1
  IN_Job/RConn1 -- start_ProcessTimer/LConn1
  ProcessServer/RConn1 -- read_ProcessTimer/LConn1
  start_ProcessTimer/RConn1 -- ProcessQueue/LConn1
  ProcessQueue/RConn1 -- ProcessServer/LConn1
  read_ProcessTimer/RConn1 -- OUTQueue/LConn1
  OUT_Job/RConn1 -- setRouting/RConn1

== system ProcessNetworkSimulation/Process_43/Process ==
  OUTQueue : FIFOQueue  Capacity=inf
  ProcessQueue : FIFOQueue  Capacity=Inf  StatAverageWait=on  StatAverageQueueLength=on
      settings: OutputPortMap=o2,o3
  ProcessServer : NServer  NumberOfServers=12  ServiceTimeFrom=Signal port t  StatNumberDeparted=on  StatUtilization=on
      settings: OutputPortMap=o0,o5
  ProcessTime : EventBasedRandomNumber  meanExp=0.05  minUnif=1  meanNorm=2  stdNorm=0.2  Seed=40488
  Routing : EventBasedRandomNumber  Distribution=Arbitrary discrete  valueVecDisc=[0,1,2,3,4,5,6,7,8,9,10,11,12,13,14,15,16,17,18,19,20,21,22,23,24,25,26,27,28,29,30,31,32,33,34,35,36,37,38,39,40,41,42]  probVecDisc=[0,0.0342,0.0256,0.0128,0.0256,0.0385,0.0043,0.0214,0.0085,0.0385,0.0085,0.0085,0.0385,0.0085,0.0256,0.0385,0.0214,0.0385,0.0385,0.0385,0.0256,0.0256,0.0342,0.0085,0.0085,0.0299,0.0299,0.0128,0.0385,0.0256,0.0085,0.043,0.0299,0.0299,0.0427,0.0214,0.0085,0.0043,0.0385,0.0085,0.0299,0.0214,0]  Seed=43705
  read_ProcessTimer : ReadTimer  TimerTag=T_Process_43  StatAverageTimeElapsed=on
      settings: OutputPortMap=o3
  setRouting : SetAttribute  AttributeName=outputFlowNode  AttributeFrom=Signal port  EvaluatedAttributeValue={ []}
  start_ProcessTimer : StartTimer  TimerTag=T_Process_43  TimerStartedOption=Restart
  IN_Job : PMIOPort  Port=1  Side=Left
  OUT_Job : PMIOPort  Port=2  Side=Right
  wires:
  Routing/1 -> setRouting/1
  ProcessTime/1 -> ProcessServer/1
  connections:
  setRouting/LConn1 -- OUTQueue/RConn1
  IN_Job/RConn1 -- start_ProcessTimer/LConn1
  ProcessServer/RConn1 -- read_ProcessTimer/LConn1
  start_ProcessTimer/RConn1 -- ProcessQueue/LConn1
  ProcessQueue/RConn1 -- ProcessServer/LConn1
  read_ProcessTimer/RConn1 -- OUTQueue/LConn1
  OUT_Job/RConn1 -- setRouting/RConn1

== system ProcessNetworkSimulation/Process_44/Process ==
  OUTQueue : FIFOQueue  Capacity=inf
  ProcessQueue : FIFOQueue  Capacity=Inf  StatAverageWait=on  StatAverageQueueLength=on
      settings: OutputPortMap=o2,o3
  ProcessServer : NServer  NumberOfServers=13  ServiceTimeFrom=Signal port t  StatNumberDeparted=on  StatUtilization=on
      settings: OutputPortMap=o0,o5
  ProcessTime : EventBasedRandomNumber  meanExp=0.05  minUnif=1  meanNorm=2  stdNorm=0.2  Seed=46922
  Routing : EventBasedRandomNumber  Distribution=Arbitrary discrete  valueVecDisc=[0,1,2,3,4,5,6,7,8,9,10,11,12,13,14,15,16,17,18,19,20,21,22,23,24,25,26,27,28,29,30,31,32,33,34,35,36,37,38,39,40,41,42,43,44,45,46]  probVecDisc=[0,0.0249,0.0214,0.0071,0.032,0.032,0.032,0.0071,0.0178,0.0071,0.0178,0.0036,0.032,0.0071,0.0214,0.032,0.032,0.032,0.0249,0.0107,0.0178,0.0249,0.0107,0.0036,0.0071,0.032,0.0214,0.0249,0.032,0.0249,0.032,0.0071,0.0071,0.032,0.0249,0.0285,0.0107,0.0358,0.032,0.032,0.0356,0.032,0.0249,0.0249,0.0249,0.0214,0]  Seed=50139
  read_ProcessTimer : ReadTimer  TimerTag=T_Process_44  StatAverageTimeElapsed=on
      settings: OutputPortMap=o3
  setRouting : SetAttribute  AttributeName=outputFlowNode  AttributeFrom=Signal port  EvaluatedAttributeValue={ []}
  start_ProcessTimer : StartTimer  TimerTag=T_Process_44  TimerStartedOption=Restart
  IN_Job : PMIOPort  Port=1  Side=Left
  OUT_Job : PMIOPort  Port=2  Side=Right
  wires:
  Routing/1 -> setRouting/1
  ProcessTime/1 -> ProcessServer/1
  connections:
  setRouting/LConn1 -- OUTQueue/RConn1
  IN_Job/RConn1 -- start_ProcessTimer/LConn1
  ProcessServer/RConn1 -- read_ProcessTimer/LConn1
  start_ProcessTimer/RConn1 -- ProcessQueue/LConn1
  ProcessQueue/RConn1 -- ProcessServer/LConn1
  read_ProcessTimer/RConn1 -- OUTQueue/LConn1
  OUT_Job/RConn1 -- setRouting/RConn1

== system ProcessNetworkSimulation/Process_45/Process ==
  OUTQueue : FIFOQueue  Capacity=inf
  ProcessQueue : FIFOQueue  Capacity=Inf  StatAverageWait=on  StatAverageQueueLength=on
      settings: OutputPortMap=o2,o3
  ProcessServer : NServer  NumberOfServers=12  ServiceTimeFrom=Signal port t  StatNumberDeparted=on  StatUtilization=on
      settings: OutputPortMap=o0,o5
  ProcessTime : EventBasedRandomNumber  meanExp=0.05  minUnif=1  meanNorm=2  stdNorm=0.2  Seed=53356
  Routing : EventBasedRandomNumber  Distribution=Arbitrary discrete  valueVecDisc=[0,1,2,3,4,5,6,7,8,9,10,11,12,13,14,15,16,17,18,19,20,21,22,23,24,25,26,27,28,29,30,31,32,33,34,35,36]  probVecDisc=[0,0.0105,0.0368,0.0368,0.0421,0.0316,0.0263,0.0053,0.0105,0.0316,0.0316,0.0368,0.0263,0.0368,0.0526,0.0316,0.0421,0.0053,0.0105,0.0158,0.0474,0.0158,0.0053,0.0474,0.0105,0.0105,0.0368,0.0421,0.0474,0.0474,0.0421,0.0158,0.0474,0.0158,0.0053,0.0421,0]  Seed=56573
  read_ProcessTimer : ReadTimer  TimerTag=T_Process_45  StatAverageTimeElapsed=on
      settings: OutputPortMap=o3
  setRouting : SetAttribute  AttributeName=outputFlowNode  AttributeFrom=Signal port  EvaluatedAttributeValue={ []}
  start_ProcessTimer : StartTimer  TimerTag=T_Process_45  TimerStartedOption=Restart
  IN_Job : PMIOPort  Port=1  Side=Left
  OUT_Job : PMIOPort  Port=2  Side=Right
  wires:
  Routing/1 -> setRouting/1
  ProcessTime/1 -> ProcessServer/1
  connections:
  setRouting/LConn1 -- OUTQueue/RConn1
  IN_Job/RConn1 -- start_ProcessTimer/LConn1
  ProcessServer/RConn1 -- read_ProcessTimer/LConn1
  start_ProcessTimer/RConn1 -- ProcessQueue/LConn1
  ProcessQueue/RConn1 -- ProcessServer/LConn1
  read_ProcessTimer/RConn1 -- OUTQueue/LConn1
  OUT_Job/RConn1 -- setRouting/RConn1

== system ProcessNetworkSimulation/Process_46/Process ==
  OUTQueue : FIFOQueue  Capacity=inf
  ProcessQueue : FIFOQueue  Capacity=Inf  StatAverageWait=on  StatAverageQueueLength=on
      settings: OutputPortMap=o2,o3
  ProcessServer : NServer  NumberOfServers=12  ServiceTimeFrom=Signal port t  StatNumberDeparted=on  StatUtilization=on
      settings: OutputPortMap=o0,o5
  ProcessTime : EventBasedRandomNumber  meanExp=0.05  minUnif=1  meanNorm=2  stdNorm=0.2  Seed=59790
  Routing : EventBasedRandomNumber  Distribution=Arbitrary discrete  valueVecDisc=[0,1,2,3,4,5,6,7,8,9,10,11,12,13,14,15,16,17,18,19,20,21,22,23,24,25,26,27,28,29,30,31,32,33,34,35,36,37,38,39,40,41]  probVecDisc=[0,0.0369,0.0276,0.0415,0.0092,0.0138,0.023,0.023,0.0323,0.0092,0.0138,0.0463,0.0276,0.0369,0.0415,0.0415,0.0092,0.0415,0.0092,0.0323,0.0138,0.0276,0.0323,0.0461,0.023,0.0323,0.0092,0.0092,0.0092,0.0323,0.023,0.0323,0.0323,0.0138,0.0323,0.023,0.0276,0.0276,0.0138,0.0138,0.0092,0]  Seed=63007
  read_ProcessTimer : ReadTimer  TimerTag=T_Process_46  StatAverageTimeElapsed=on
      settings: OutputPortMap=o3
  setRouting : SetAttribute  AttributeName=outputFlowNode  AttributeFrom=Signal port  EvaluatedAttributeValue={ []}
  start_ProcessTimer : StartTimer  TimerTag=T_Process_46  TimerStartedOption=Restart
  IN_Job : PMIOPort  Port=1  Side=Left
  OUT_Job : PMIOPort  Port=2  Side=Right
  wires:
  Routing/1 -> setRouting/1
  ProcessTime/1 -> ProcessServer/1
  connections:
  setRouting/LConn1 -- OUTQueue/RConn1
  IN_Job/RConn1 -- start_ProcessTimer/LConn1
  ProcessServer/RConn1 -- read_ProcessTimer/LConn1
  start_ProcessTimer/RConn1 -- ProcessQueue/LConn1
  ProcessQueue/RConn1 -- ProcessServer/LConn1
  read_ProcessTimer/RConn1 -- OUTQueue/LConn1
  OUT_Job/RConn1 -- setRouting/RConn1

== system ProcessNetworkSimulation/Process_47/Process ==
  OUTQueue : FIFOQueue  Capacity=inf
  ProcessQueue : FIFOQueue  Capacity=Inf  StatAverageWait=on  StatAverageQueueLength=on
      settings: OutputPortMap=o2,o3
  ProcessServer : NServer  NumberOfServers=12  ServiceTimeFrom=Signal port t  StatNumberDeparted=on  StatUtilization=on
      settings: OutputPortMap=o0,o5
  ProcessTime : EventBasedRandomNumber  meanExp=0.05  minUnif=1  meanNorm=2  stdNorm=0.2  Seed=688
  Routing : EventBasedRandomNumber  Distribution=Arbitrary discrete  valueVecDisc=[0,1,2,3,4,5,6,7,8,9,10,11,12,13,14,15,16,17,18,19,20,21,22,23,24,25,26,27,28,29,30,31,32,33,34]  probVecDisc=[0,0.0357,0.0459,0.0255,0.0306,0.0255,0.0255,0.0459,0.0357,0.0102,0.0514,0.051,0.0102,0.0408,0.0153,0.0357,0.0153,0.0255,0.0357,0.0459,0.0255,0.0459,0.0459,0.0102,0.0102,0.0357,0.0459,0.0102,0.0459,0.0255,0.0255,0.0102,0.0102,0.0459,0]  Seed=3905
  read_ProcessTimer : ReadTimer  TimerTag=T_Process_47  StatAverageTimeElapsed=on
      settings: OutputPortMap=o3
  setRouting : SetAttribute  AttributeName=outputFlowNode  AttributeFrom=Signal port  EvaluatedAttributeValue={ []}
  start_ProcessTimer : StartTimer  TimerTag=T_Process_47  TimerStartedOption=Restart
  IN_Job : PMIOPort  Port=1  Side=Left
  OUT_Job : PMIOPort  Port=2  Side=Right
  wires:
  Routing/1 -> setRouting/1
  ProcessTime/1 -> ProcessServer/1
  connections:
  setRouting/LConn1 -- OUTQueue/RConn1
  IN_Job/RConn1 -- start_ProcessTimer/LConn1
  ProcessServer/RConn1 -- read_ProcessTimer/LConn1
  start_ProcessTimer/RConn1 -- ProcessQueue/LConn1
  ProcessQueue/RConn1 -- ProcessServer/LConn1
  read_ProcessTimer/RConn1 -- OUTQueue/LConn1
  OUT_Job/RConn1 -- setRouting/RConn1
